simulink model "sfunction_test"  (R2014a)
settings: Solver=ode45  StartTime=0.0  StopTime=10.0  RelTol=1e-3
settings Model: Creator=scorpii  LastModifiedBy=scorpii

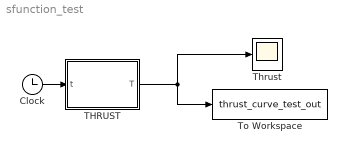
== system sfunction_test ==
  Clock : Clock
  THRUST : Subsystem  TreatAsAtomicUnit=on
  Thrust : Scope
  To Workspace : ToWorkspace  VariableName=thrust_curve_test_out  SampleTime=-1
  wires:
  Clock/1 -> THRUST/1(t)
  THRUST/1(T) -> Thrust/1, To Workspace/1

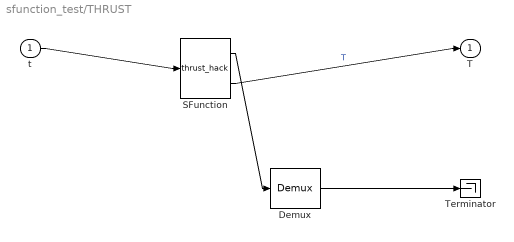
== system sfunction_test/THRUST ==
  t : Inport
  " Demux " : Demux  Outputs=1
  " SFunction " : S-Function  Tag=Stateflow S-Function VELOCITY_MODEL 2  FunctionName=thrust_hack  PortCounts=[1 2]  EnableBusSupport=on
  " Terminator " : Terminator
  T : Outport
  wires:
  t/1 -> " SFunction "/1
  " SFunction "/2 -> T/1  "T"
  " Demux "/1 -> " Terminator "/1
  " SFunction "/1 -> " Demux "/1
